simulink model "POD1_SDES"  (R2018a)
settings: Solver=ode45  StartTime=0.0  StopTime=100  RelTol=1e-3
values from neighbouring files (symbols this model uses):
  G = 9.81    [SEDS_Cascade_P1.m]
  Ix = 0.5*m*l^2    [SEDS_Cascade_P1.m]
  Iy = Ix    [SEDS_Cascade_P1.m]
  Iz = Ix + Iy    [SEDS_Cascade_P1.m]
  m = 0.053    [SEDS_Cascade_P1.m]
  wn_att = 4/(zeta_att*Tr_att)    (= 10)    [SEDS_Cascade_P1.m]
  zeta_att = 0.8    [SEDS_Cascade_P1.m]
libraries: simulink x6
settings Model: Creator=Ndeye Khady NDIAYE  LastModifiedBy=Ndeye Khady NDIAYE

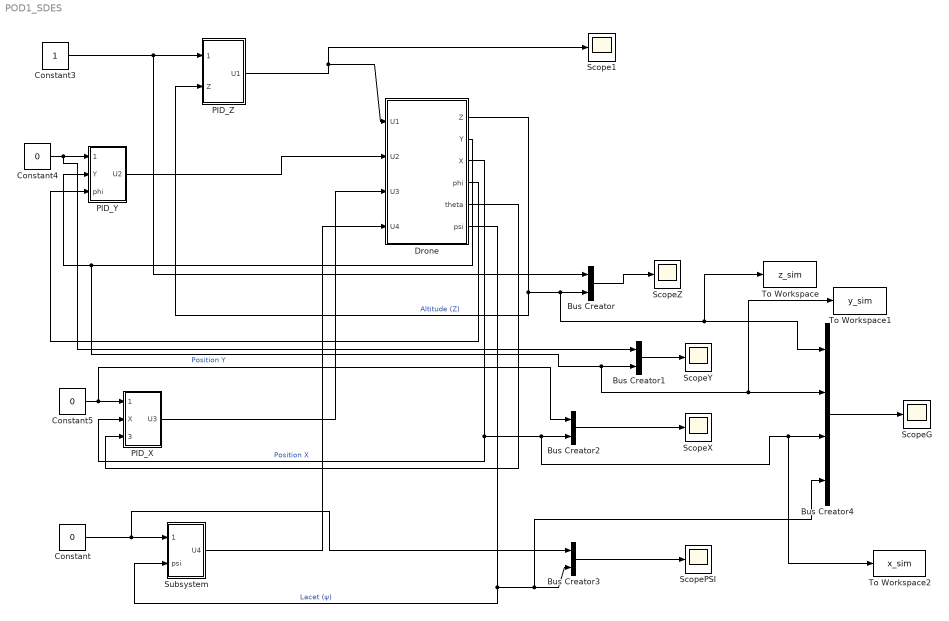
== system POD1_SDES ==
  Bus Creator{,1..3} (4 alike) : BusCreator  Inputs=2
  Bus Creator4 : BusCreator  Inputs=4
  Constant : Constant  Value=0
  Constant3 : Constant
  Constant4 : Constant  Value=0
  Constant5 : Constant  Value=0
  Drone : Subsystem
  PID_X : Subsystem
  PID_Y : Subsystem
  PID_Z : Subsystem
  Scope1 : Scope
  ScopeG : Scope
  ScopePSI : Scope
  ScopeX : Scope
  ScopeY : Scope
  ScopeZ : Scope
  Subsystem : Subsystem
  To Workspace : ToWorkspace  VariableName=z_sim  SampleTime=-1
  To Workspace1 : ToWorkspace  VariableName=y_sim  SampleTime=-1
  To Workspace2 : ToWorkspace  VariableName=x_sim  SampleTime=-1
  wires:
  Subsystem/1(U4) -> Drone/4(U4)
  Drone/6(psi) -> Bus Creator4/4, Bus Creator3/2, Subsystem/2(psi)  "Lacet (ψ)"
  PID_X/1(U3) -> Drone/3(U3)
  Bus Creator3/1 -> ScopePSI/1
  Constant3/1 -> Bus Creator/1, PID_Z/1(Z_ref)
  Drone/4(phi) -> PID_Y/3(phi)
  Bus Creator1/1 -> ScopeY/1
  Bus Creator2/1 -> ScopeX/1
  Bus Creator/1 -> ScopeZ/1
  Constant5/1 -> Bus Creator2/1, PID_X/1(X_ref)
  Drone/3(X) -> To Workspace2/1, Bus Creator4/3, Bus Creator2/2, PID_X/2(X)  "Position X"
  Drone/2(Y) -> To Workspace1/1, Bus Creator4/2, Bus Creator1/2, PID_Y/2(Y)  "Position Y"
  Drone/1(Z) -> To Workspace/1, Bus Creator4/1, Bus Creator/2, PID_Z/2(Z)  "Altitude (Z)"
  PID_Y/1(U2) -> Drone/2(U2)
  Constant/1 -> Bus Creator3/1, Subsystem/1(psi_ref)
  Constant4/1 -> Bus Creator1/1, PID_Y/1(Y_ref)
  Drone/5(theta) -> PID_X/3(theta)
  PID_Z/1("U1 ") -> Scope1/1, Drone/1(U1)
  Bus Creator4/1 -> ScopeG/1

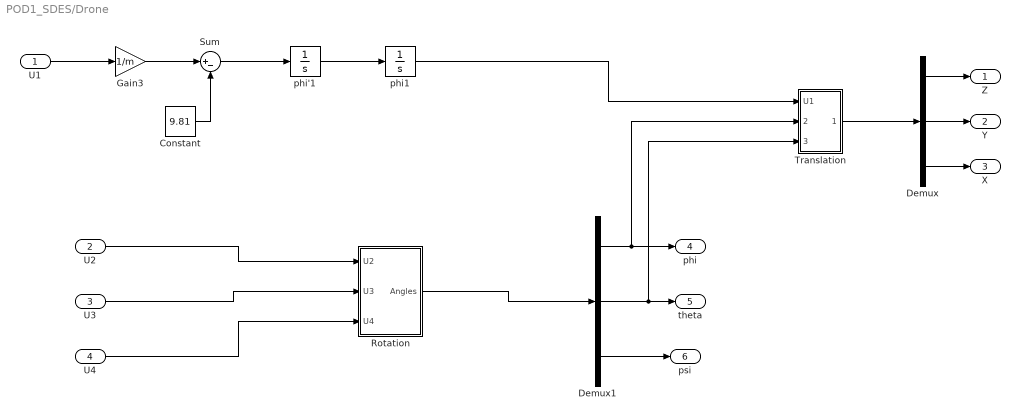
== system POD1_SDES/Drone ==
  U1 : Inport
  U2 : Inport  Port=2
  U3 : Inport  Port=3
  U4 : Inport  Port=4
  Constant : Constant  Value=9.81
  Demux : Demux  Outputs=3
  Demux1 : Demux  Outputs=3
  Gain3 : Gain  Gain=1/m
  Rotation : Subsystem
  Sum : Sum  Inputs=|+-
  Translation : Subsystem
  phi'1 : Integrator
  phi1 : Integrator
  Z : Outport
  Y : Outport  Port=2
  X : Outport  Port=3
  phi : Outport  Port=4
  theta : Outport  Port=5
  psi : Outport  Port=6
  wires:
  Sum/1 -> phi'1/1
  phi'1/1 -> phi1/1
  Gain3/1 -> Sum/1
  U1/1 -> Gain3/1
  Constant/1 -> Sum/2
  phi1/1 -> Translation/1(U1)
  Translation/1(ZYX) -> Demux/1
  Demux/1 -> Z/1
  Demux/2 -> Y/1
  Demux/3 -> X/1
  U2/1 -> Rotation/1(U2)
  U3/1 -> Rotation/2(U3)
  U4/1 -> Rotation/3(U4)
  Rotation/1(Angles) -> Demux1/1
  Demux1/1 -> Translation/2(phi), phi/1
  Demux1/2 -> Translation/3(theta), theta/1
  Demux1/3 -> psi/1

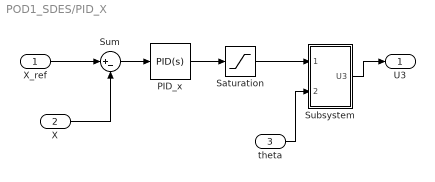
== system POD1_SDES/PID_X ==
  X_ref : Inport
  X : Inport  Port=2
  theta : Inport  Port=3
  PID_x : simulink/Continuous/PID Controller  Controller=PID  TimeDomain=Continuous-time  SampleTime=-1  IntegratorMethod=Forward Euler  FilterMethod=Forward Euler  Form=Parallel  UseFilter=on  ControllerParametersSource=internal  P=0.10  I=5e-4  D=0.14  N=50  InitialConditionSource=internal  InitialConditionForIntegrator=0  InitialConditionForFilter=0  ExternalReset=none  LimitOutput=off  UpperSaturationLimit=inf  LowerSaturationLimit=-inf  LinearizeAsGain=on  AntiWindupMode=none  Kb=1  TrackingMode=off  Kt=1  PParamMin=[]  PParamMax=[]  IParamMin=[]  IParamMax=[]  DParamMin=[]  DParamMax=[]  NParamMin=[]  NParamMax=[]  KbParamMin=[]  KbParamMax=[]  KtParamMin=[]  KtParamMax=[]  POutMin=[]  POutMax=[]  IOutMin=[]  IOutMax=[]  DOutMin=[]  DOutMax=[]  NOutMin=[]  NOutMax=[]  KbOutMin=[]  KbOutMax=[]  KtOutMin=[]  KtOutMax=[]  IntegratorOutMin=[]  IntegratorOutMax=[]  FilterOutMin=[]  FilterOutMax=[]  SumOutMin=[]  SumOutMax=[]  SumI1OutMin=[]  SumI1OutMax=[]  SumI2OutMin=[]  SumI2OutMax=[]  SumI3OutMin=[]  SumI3OutMax=[]  SumDOutMin=[]  SumDOutMax=[]  SaturationOutMin=[]  SaturationOutMax=[]  IntegratorContinuousStateAttributes=''  IntegratorStateMustResolveToSignalObject=off  IntegratorRTWStateStorageClass=Auto  FilterContinuousStateAttributes=''  FilterStateMustResolveToSignalObject=off  FilterRTWStateStorageClass=Auto  DifferentiatorICPrevScaledInput=0  DifferentiatorOutMin=[]  DifferentiatorOutMax=[]  FilterDiffOutCoefMin=[]  FilterDiffOutCoefMax=[]  SumDenOutMin=[]  SumDenOutMax=[]  SumNumOutMin=[]  SumNumOutMax=[]  ReciprocalOutMin=[]  ReciprocalOutMax=[]  DivideOutMin=[]  DivideOutMax=[]  TunerSelectOption=Transfer Function Based (PID Tuner App)
  Saturation : Saturate  UpperLimit=0.25  LowerLimit=-0.25
  Subsystem : Subsystem
  Sum : Sum  Inputs=|+-
  U3 : Outport
  wires:
  X/1 -> Sum/2
  X_ref/1 -> Sum/1
  Sum/1 -> PID_x/1
  Subsystem/1(U3) -> U3/1
  theta/1 -> Subsystem/2(theta)
  PID_x/1 -> Saturation/1
  Saturation/1 -> Subsystem/1(theta_ref)

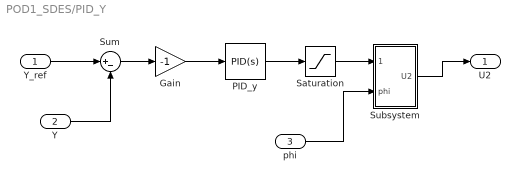
== system POD1_SDES/PID_Y ==
  Y_ref : Inport
  Y : Inport  Port=2
  phi : Inport  Port=3
  Gain : Gain  Gain=-1
  PID_y : simulink/Continuous/PID Controller  Controller=PID  TimeDomain=Continuous-time  SampleTime=-1  IntegratorMethod=Forward Euler  FilterMethod=Forward Euler  Form=Parallel  UseFilter=on  ControllerParametersSource=internal  P=0.10  I=5e-4  D=0.14  N=50  InitialConditionSource=internal  InitialConditionForIntegrator=0  InitialConditionForFilter=0  ExternalReset=none  LimitOutput=on  UpperSaturationLimit=inf  LowerSaturationLimit=-inf  LinearizeAsGain=on  AntiWindupMode=clamping  Kb=1  TrackingMode=off  Kt=1  PParamMin=[]  PParamMax=[]  IParamMin=[]  IParamMax=[]  DParamMin=[]  DParamMax=[]  NParamMin=[]  NParamMax=[]  KbParamMin=[]  KbParamMax=[]  KtParamMin=[]  KtParamMax=[]  POutMin=[]  POutMax=[]  IOutMin=[]  IOutMax=[]  DOutMin=[]  DOutMax=[]  NOutMin=[]  NOutMax=[]  KbOutMin=[]  KbOutMax=[]  KtOutMin=[]  KtOutMax=[]  IntegratorOutMin=[]  IntegratorOutMax=[]  FilterOutMin=[]  FilterOutMax=[]  SumOutMin=[]  SumOutMax=[]  SumI1OutMin=[]  SumI1OutMax=[]  SumI2OutMin=[]  SumI2OutMax=[]  SumI3OutMin=[]  SumI3OutMax=[]  SumDOutMin=[]  SumDOutMax=[]  SaturationOutMin=[]  SaturationOutMax=[]  IntegratorContinuousStateAttributes=''  IntegratorStateMustResolveToSignalObject=off  IntegratorRTWStateStorageClass=Auto  FilterContinuousStateAttributes=''  FilterStateMustResolveToSignalObject=off  FilterRTWStateStorageClass=Auto  DifferentiatorICPrevScaledInput=0  DifferentiatorOutMin=[]  DifferentiatorOutMax=[]  FilterDiffOutCoefMin=[]  FilterDiffOutCoefMax=[]  SumDenOutMin=[]  SumDenOutMax=[]  SumNumOutMin=[]  SumNumOutMax=[]  ReciprocalOutMin=[]  ReciprocalOutMax=[]  DivideOutMin=[]  DivideOutMax=[]  TunerSelectOption=Transfer Function Based (PID Tuner App)
  Saturation : Saturate  UpperLimit=0.25  LowerLimit=-0.25
  Subsystem : Subsystem
  Sum : Sum  Inputs=|+-
  U2 : Outport
  wires:
  Y/1 -> Sum/2
  Y_ref/1 -> Sum/1
  Subsystem/1(U2) -> U2/1
  phi/1 -> Subsystem/2(phi)
  PID_y/1 -> Saturation/1
  Saturation/1 -> Subsystem/1(phi_ref)
  Sum/1 -> Gain/1
  Gain/1 -> PID_y/1

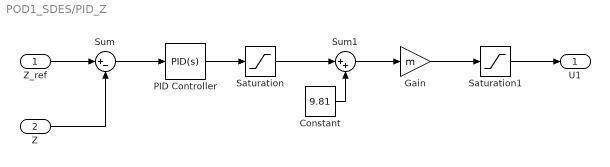
== system POD1_SDES/PID_Z ==
  Z_ref : Inport
  Z : Inport  Port=2
  Constant : Constant  Value=9.81
  Gain : Gain  Gain=m
  PID Controller : simulink/Continuous/PID Controller  Controller=PID  TimeDomain=Continuous-time  SampleTime=-1  IntegratorMethod=Forward Euler  FilterMethod=Forward Euler  Form=Parallel  UseFilter=on  ControllerParametersSource=internal  P=16  I=0.005  D=7.0  N=50  InitialConditionSource=internal  InitialConditionForIntegrator=0  InitialConditionForFilter=0  ExternalReset=none  LimitOutput=on  UpperSaturationLimit=inf  LowerSaturationLimit=-inf  LinearizeAsGain=on  AntiWindupMode=clamping  Kb=1  TrackingMode=off  Kt=1  PParamMin=[]  PParamMax=[]  IParamMin=[]  IParamMax=[]  DParamMin=[]  DParamMax=[]  NParamMin=[]  NParamMax=[]  KbParamMin=[]  KbParamMax=[]  KtParamMin=[]  KtParamMax=[]  POutMin=[]  POutMax=[]  IOutMin=[]  IOutMax=[]  DOutMin=[]  DOutMax=[]  NOutMin=[]  NOutMax=[]  KbOutMin=[]  KbOutMax=[]  KtOutMin=[]  KtOutMax=[]  IntegratorOutMin=[]  IntegratorOutMax=[]  FilterOutMin=[]  FilterOutMax=[]  SumOutMin=[]  SumOutMax=[]  SumI1OutMin=[]  SumI1OutMax=[]  SumI2OutMin=[]  SumI2OutMax=[]  SumI3OutMin=[]  SumI3OutMax=[]  SumDOutMin=[]  SumDOutMax=[]  SaturationOutMin=[]  SaturationOutMax=[]  IntegratorContinuousStateAttributes=''  IntegratorStateMustResolveToSignalObject=off  IntegratorRTWStateStorageClass=Auto  FilterContinuousStateAttributes=''  FilterStateMustResolveToSignalObject=off  FilterRTWStateStorageClass=Auto  DifferentiatorICPrevScaledInput=0  DifferentiatorOutMin=[]  DifferentiatorOutMax=[]  FilterDiffOutCoefMin=[]  FilterDiffOutCoefMax=[]  SumDenOutMin=[]  SumDenOutMax=[]  SumNumOutMin=[]  SumNumOutMax=[]  ReciprocalOutMin=[]  ReciprocalOutMax=[]  DivideOutMin=[]  DivideOutMax=[]  TunerSelectOption=Transfer Function Based (PID Tuner App)
  Saturation : Saturate  UpperLimit=19.62  LowerLimit=-9.81
  Saturation1 : Saturate  UpperLimit=3*m*G  LowerLimit=0
  Sum : Sum  Inputs=|+-
  Sum1 : Sum  Inputs=|++
  "U1 " : Outport
  wires:
  PID Controller/1 -> Saturation/1
  Z_ref/1 -> Sum/1
  Sum/1 -> PID Controller/1
  Z/1 -> Sum/2
  Saturation/1 -> Sum1/1
  Sum1/1 -> Gain/1
  Constant/1 -> Sum1/2
  Gain/1 -> Saturation1/1
  Saturation1/1 -> "U1 "/1

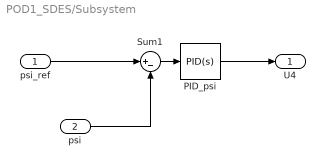
== system POD1_SDES/Subsystem ==
  psi_ref : Inport
  psi : Inport  Port=2
  PID_psi : simulink/Continuous/PID Controller  Controller=PID  TimeDomain=Continuous-time  SampleTime=-1  IntegratorMethod=Forward Euler  FilterMethod=Forward Euler  Form=Parallel  UseFilter=on  ControllerParametersSource=internal  P=Iz*wn_att^2  I=0.005  D=2*zeta_att*Iz*wn_att  N=50  InitialConditionSource=internal  InitialConditionForIntegrator=0  InitialConditionForFilter=0  ExternalReset=none  LimitOutput=off  UpperSaturationLimit=inf  LowerSaturationLimit=-inf  LinearizeAsGain=on  AntiWindupMode=none  Kb=1  TrackingMode=off  Kt=1  PParamMin=[]  PParamMax=[]  IParamMin=[]  IParamMax=[]  DParamMin=[]  DParamMax=[]  NParamMin=[]  NParamMax=[]  KbParamMin=[]  KbParamMax=[]  KtParamMin=[]  KtParamMax=[]  POutMin=[]  POutMax=[]  IOutMin=[]  IOutMax=[]  DOutMin=[]  DOutMax=[]  NOutMin=[]  NOutMax=[]  KbOutMin=[]  KbOutMax=[]  KtOutMin=[]  KtOutMax=[]  IntegratorOutMin=[]  IntegratorOutMax=[]  FilterOutMin=[]  FilterOutMax=[]  SumOutMin=[]  SumOutMax=[]  SumI1OutMin=[]  SumI1OutMax=[]  SumI2OutMin=[]  SumI2OutMax=[]  SumI3OutMin=[]  SumI3OutMax=[]  SumDOutMin=[]  SumDOutMax=[]  SaturationOutMin=[]  SaturationOutMax=[]  IntegratorContinuousStateAttributes=''  IntegratorStateMustResolveToSignalObject=off  IntegratorRTWStateStorageClass=Auto  FilterContinuousStateAttributes=''  FilterStateMustResolveToSignalObject=off  FilterRTWStateStorageClass=Auto  DifferentiatorICPrevScaledInput=0  DifferentiatorOutMin=[]  DifferentiatorOutMax=[]  FilterDiffOutCoefMin=[]  FilterDiffOutCoefMax=[]  SumDenOutMin=[]  SumDenOutMax=[]  SumNumOutMin=[]  SumNumOutMax=[]  ReciprocalOutMin=[]  ReciprocalOutMax=[]  DivideOutMin=[]  DivideOutMax=[]  TunerSelectOption=Transfer Function Based (PID Tuner App)
  Sum1 : Sum  Inputs=|+-
  U4 : Outport
  wires:
  Sum1/1 -> PID_psi/1
  psi/1 -> Sum1/2
  psi_ref/1 -> Sum1/1
  PID_psi/1 -> U4/1

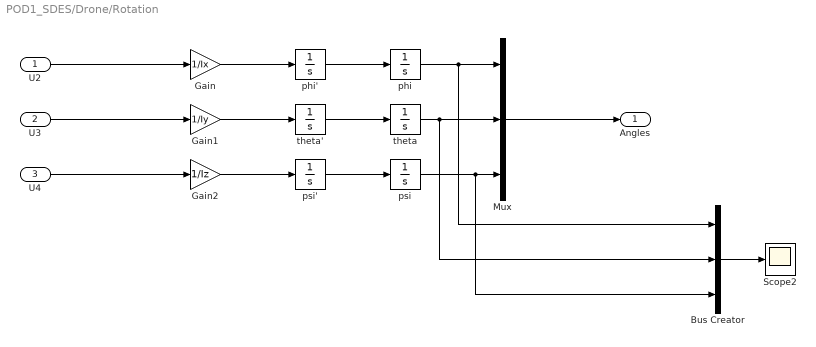
== system POD1_SDES/Drone/Rotation ==
  U2 : Inport
  U3 : Inport  Port=2
  U4 : Inport  Port=3
  Bus Creator : BusCreator  Inputs=3
  Gain : Gain  Gain=1/Ix
  Gain1 : Gain  Gain=1/Iy
  Gain2 : Gain  Gain=1/Iz
  Mux : Mux  Inputs=3
  Scope2 : Scope
  phi : Integrator
  phi' : Integrator
  psi : Integrator
  psi' : Integrator
  theta : Integrator
  theta' : Integrator
  Angles : Outport
  wires:
  phi/1 -> Bus Creator/1, Mux/1
  psi'/1 -> psi/1
  theta'/1 -> theta/1
  Gain2/1 -> psi'/1
  phi'/1 -> phi/1
  psi/1 -> Bus Creator/3, Mux/3
  theta/1 -> Bus Creator/2, Mux/2
  Gain/1 -> phi'/1
  Gain1/1 -> theta'/1
  U3/1 -> Gain1/1
  Mux/1 -> Angles/1
  U4/1 -> Gain2/1
  U2/1 -> Gain/1
  Bus Creator/1 -> Scope2/1

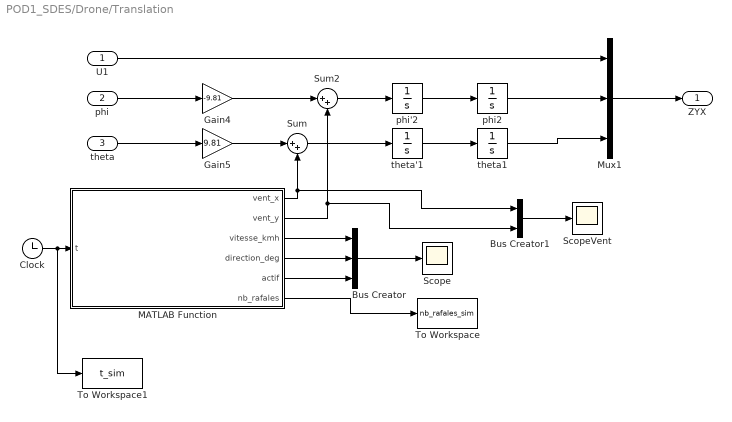
== system POD1_SDES/Drone/Translation ==
  U1 : Inport
  phi : Inport  Port=2
  theta : Inport  Port=3
  Bus Creator : BusCreator  Inputs=3
  Bus Creator1 : BusCreator  Inputs=2
  Clock : Clock
  Gain4 : Gain  Gain=-9.81
  Gain5 : Gain  Gain=9.81
  MATLAB Function : MATLAB Function  TreatAsAtomicUnit=on
  Mux1 : Mux  Inputs=3
  Scope : Scope
  ScopeVent : Scope
  Sum : Sum  Inputs=|++
  Sum2 : Sum  Inputs=|++
  To Workspace : ToWorkspace  VariableName=nb_rafales_sim  SampleTime=-1
  To Workspace1 : ToWorkspace  VariableName=t_sim  SampleTime=-1
  phi'2 : Integrator
  phi2 : Integrator
  theta'1 : Integrator
  theta1 : Integrator
  ZYX : Outport
  wires:
  Mux1/1 -> ZYX/1
  phi'2/1 -> phi2/1
  theta'1/1 -> theta1/1
  theta/1 -> Gain5/1
  U1/1 -> Mux1/1
  theta1/1 -> Mux1/3
  phi2/1 -> Mux1/2
  phi/1 -> Gain4/1
  Gain5/1 -> Sum/1
  Sum/1 -> theta'1/1
  Gain4/1 -> Sum2/1
  Sum2/1 -> phi'2/1
  Clock/1 -> To Workspace1/1, MATLAB Function/1(t)
  MATLAB Function/2(vent_y) -> Bus Creator1/2, Sum2/2
  MATLAB Function/1(vent_x) -> Bus Creator1/1, Sum/2
  MATLAB Function/6(nb_rafales) -> To Workspace/1
  MATLAB Function/3(vitesse_kmh) -> Bus Creator/1
  MATLAB Function/4(direction_deg) -> Bus Creator/2
  MATLAB Function/5(actif) -> Bus Creator/3
  Bus Creator/1 -> Scope/1
  Bus Creator1/1 -> ScopeVent/1

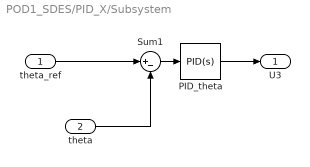
== system POD1_SDES/PID_X/Subsystem ==
  theta_ref : Inport
  theta : Inport  Port=2
  PID_theta : simulink/Continuous/PID Controller  Controller=PID  TimeDomain=Continuous-time  SampleTime=-1  IntegratorMethod=Forward Euler  FilterMethod=Forward Euler  Form=Parallel  UseFilter=on  ControllerParametersSource=internal  P=Iy*wn_att^2  I=0.005  D=2*zeta_att*Iy*wn_att  N=100  InitialConditionSource=internal  InitialConditionForIntegrator=0  InitialConditionForFilter=0  ExternalReset=none  LimitOutput=off  UpperSaturationLimit=inf  LowerSaturationLimit=-inf  LinearizeAsGain=on  AntiWindupMode=none  Kb=1  TrackingMode=off  Kt=1  PParamMin=[]  PParamMax=[]  IParamMin=[]  IParamMax=[]  DParamMin=[]  DParamMax=[]  NParamMin=[]  NParamMax=[]  KbParamMin=[]  KbParamMax=[]  KtParamMin=[]  KtParamMax=[]  POutMin=[]  POutMax=[]  IOutMin=[]  IOutMax=[]  DOutMin=[]  DOutMax=[]  NOutMin=[]  NOutMax=[]  KbOutMin=[]  KbOutMax=[]  KtOutMin=[]  KtOutMax=[]  IntegratorOutMin=[]  IntegratorOutMax=[]  FilterOutMin=[]  FilterOutMax=[]  SumOutMin=[]  SumOutMax=[]  SumI1OutMin=[]  SumI1OutMax=[]  SumI2OutMin=[]  SumI2OutMax=[]  SumI3OutMin=[]  SumI3OutMax=[]  SumDOutMin=[]  SumDOutMax=[]  SaturationOutMin=[]  SaturationOutMax=[]  IntegratorContinuousStateAttributes=''  IntegratorStateMustResolveToSignalObject=off  IntegratorRTWStateStorageClass=Auto  FilterContinuousStateAttributes=''  FilterStateMustResolveToSignalObject=off  FilterRTWStateStorageClass=Auto  DifferentiatorICPrevScaledInput=0  DifferentiatorOutMin=[]  DifferentiatorOutMax=[]  FilterDiffOutCoefMin=[]  FilterDiffOutCoefMax=[]  SumDenOutMin=[]  SumDenOutMax=[]  SumNumOutMin=[]  SumNumOutMax=[]  ReciprocalOutMin=[]  ReciprocalOutMax=[]  DivideOutMin=[]  DivideOutMax=[]  TunerSelectOption=Transfer Function Based (PID Tuner App)
  Sum1 : Sum  Inputs=|+-
  U3 : Outport
  wires:
  Sum1/1 -> PID_theta/1
  PID_theta/1 -> U3/1
  theta_ref/1 -> Sum1/1
  theta/1 -> Sum1/2

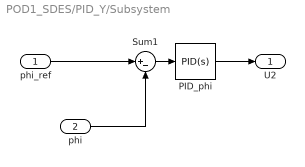
== system POD1_SDES/PID_Y/Subsystem ==
  phi_ref : Inport
  phi : Inport  Port=2
  PID_phi : simulink/Continuous/PID Controller  Controller=PID  TimeDomain=Continuous-time  SampleTime=-1  IntegratorMethod=Forward Euler  FilterMethod=Forward Euler  Form=Parallel  UseFilter=on  ControllerParametersSource=internal  P=Ix*wn_att^2  I=0.005  D=2*zeta_att*Ix*wn_att  N=50  InitialConditionSource=internal  InitialConditionForIntegrator=0  InitialConditionForFilter=0  ExternalReset=none  LimitOutput=on  UpperSaturationLimit=inf  LowerSaturationLimit=-inf  LinearizeAsGain=on  AntiWindupMode=clamping  Kb=1  TrackingMode=off  Kt=1  PParamMin=[]  PParamMax=[]  IParamMin=[]  IParamMax=[]  DParamMin=[]  DParamMax=[]  NParamMin=[]  NParamMax=[]  KbParamMin=[]  KbParamMax=[]  KtParamMin=[]  KtParamMax=[]  POutMin=[]  POutMax=[]  IOutMin=[]  IOutMax=[]  DOutMin=[]  DOutMax=[]  NOutMin=[]  NOutMax=[]  KbOutMin=[]  KbOutMax=[]  KtOutMin=[]  KtOutMax=[]  IntegratorOutMin=[]  IntegratorOutMax=[]  FilterOutMin=[]  FilterOutMax=[]  SumOutMin=[]  SumOutMax=[]  SumI1OutMin=[]  SumI1OutMax=[]  SumI2OutMin=[]  SumI2OutMax=[]  SumI3OutMin=[]  SumI3OutMax=[]  SumDOutMin=[]  SumDOutMax=[]  SaturationOutMin=[]  SaturationOutMax=[]  IntegratorContinuousStateAttributes=''  IntegratorStateMustResolveToSignalObject=off  IntegratorRTWStateStorageClass=Auto  FilterContinuousStateAttributes=''  FilterStateMustResolveToSignalObject=off  FilterRTWStateStorageClass=Auto  DifferentiatorICPrevScaledInput=0  DifferentiatorOutMin=[]  DifferentiatorOutMax=[]  FilterDiffOutCoefMin=[]  FilterDiffOutCoefMax=[]  SumDenOutMin=[]  SumDenOutMax=[]  SumNumOutMin=[]  SumNumOutMax=[]  ReciprocalOutMin=[]  ReciprocalOutMax=[]  DivideOutMin=[]  DivideOutMax=[]  TunerSelectOption=Transfer Function Based (PID Tuner App)
  Sum1 : Sum  Inputs=|+-
  U2 : Outport
  wires:
  Sum1/1 -> PID_phi/1
  PID_phi/1 -> U2/1
  phi_ref/1 -> Sum1/1
  phi/1 -> Sum1/2

== matlab function POD1_SDES/Drone/Translation/MATLAB Function ==
  settings: updateMethod=DISCRETE
  data: t input; vent_x output; vent_y output; vitesse_kmh output; direction_deg output; actif output; nb_rafales output
function [vent_x, vent_y, vitesse_kmh, direction_deg, actif, nb_rafales] = Generateur_Rafales(t)

persistent active t_start duree vitesse direction t_next compteur

if isempty(active)

    active = false;
    t_start = 0;
    duree = 0;
    vitesse = 0;
    direction = 0;
    t_next = 2 + 2*rand;

    compteur = 0;

end

vent_x = 0;
vent_y = 0;
vitesse_kmh = 0;
direction_deg = 0;
actif = 0;
nb_rafales = compteur;

if (~active) && (t >= t_next)

    active = true;
    compteur = compteur + 1;

    t_start = t;

    duree = 1 + 3*rand;        % duree entre 1 et 4 s
    vitesse = 2 + 8*rand;      % vitesse entre 2 et 10 km/h
    direction = 360*rand;      % direction entre 0 et 360 deg

end

if active && ((t - t_start) >= duree)

    active = false;
    t_next = t + 2 + 3*rand;   % prochaine rafale entre 2 et 5 s

end

if active

    coeff = 0.015;

    vent_x = coeff * vitesse * cosd(direction);
    vent_y = coeff * vitesse * sind(direction);

    vitesse_kmh = vitesse;
    direction_deg = direction;
    actif = 1;

end

nb_rafales = compteur;

end
